simulink model "Battery_Model"  (R2019b)
settings: configuration reference "BMS_Sw_CodeGenConfig" (kept outside this file)
undefined symbols (not defined in the file): Battery, TempInit, ts
libraries: fl_lib x2765, nesl_utility x1565, ee_lib x384, simulink x384, BatteryPack_lib x3
(part 1 of 33)
settings Model: DataDictionary=DD_Battery.sldd  EnableAccessToBaseWorkspace=off  Creator=mluethy  LastModifiedBy=ZHOU Jinhan
settings ConfigSetRef: SourceName=BMS_Sw_CodeGenConfig

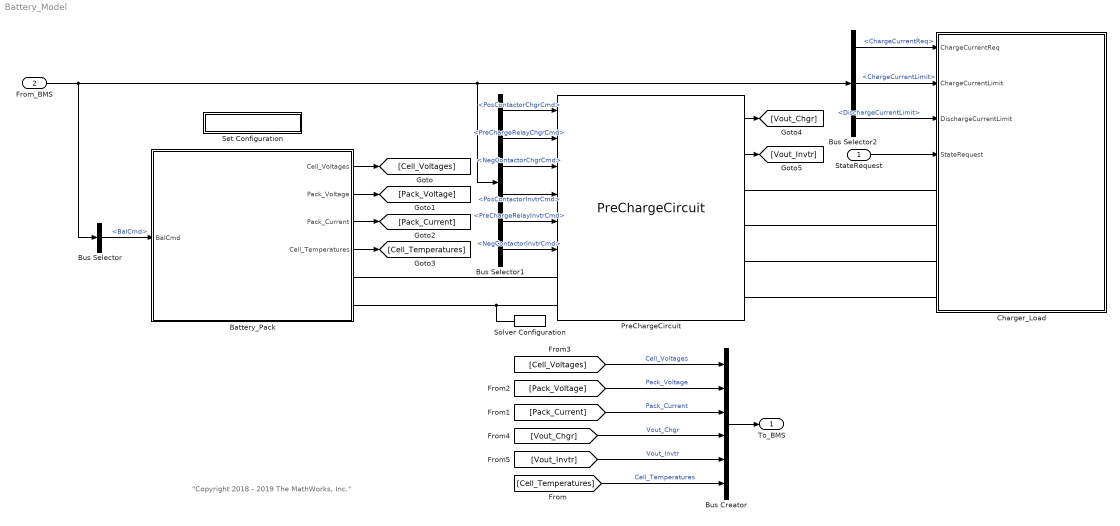
== system Battery_Model ==
  note: "Copyright 2018 - 2019 The MathWorks, Inc."
  StateRequest : Inport  OutDataTypeStr=Enum: SRE  SampleTime=[ts,0]  Interpolate=off
  From_BMS : Inport  Port=2  OutDataTypeStr=Bus: BMS_Output
  Battery_Pack : Subsystem  Variant=on  VariantControl=Variant1
      mask Display: image('Plant_Battery.jpg',[40,65,120,70])
  Bus Selector : BusSelector  OutputSignals=BalCmd
  Bus Selector1 : BusSelector  OutputSignals=PosContactorChgrCmd,PreChargeRelayChgrCmd,NegContactorChgrCmd,PosContactorInvtrCmd,PreChargeRelayInvtrCmd,NegContactorInvtrCmd
  Bus Selector2 : BusSelector  OutputSignals=ChargeCurrentReq,ChargeCurrentLimit,DischargeCurrentLimit
  Bus Creator : BusCreator  Inputs=6  OutDataTypeStr=Bus: BMS_Input  NonVirtualBus=on
  Charger_Load : Subsystem
      mask Display: image('Charger_Load3.jpg',[40,5,150,200])
  PreChargeCircuit : BatteryPack_lib/PreChargeCircuit  SystemSampleTime=-1  Latency=0  AutoFrameSizeCalculation=off
      mask Display: image('PowerElectronics.jpg',[110,60,100,100])
  Set Configuration : Subsystem
      mask Display: disp('Set Plant Configuration');
  Solver Configuration : nesl_utility/Solver Configuration  PhysicalDomain=network_engine_domain  SubClassName=solver  LeftPortType=input  RightPortType=generic  Tones=[]  Harmonics=[]  SimulateNoise=off  Profile=off  UseLocalSampling=off  EnableSwitchedLinearOptims=on  FrequencyDomain=off  UseCCode=off  RelTol=0.001  AbsTol=1e-06  MinStep=1e-09  ToWorkspace=off  RevertToSquareIcSolve=off  NumHomotopyIterations=100  PhasorMode=off  PhasorModeNumHarmonics=1  DoDC=off  ResidualTolerance=1e-09  UseLocalSolver=on  LocalSolverChoice=NE_BACKWARD_EULER_ADVANCER  LocalSolverSampleTime=ts  DoFixedCost=on  MaxNonlinIter=3  MaxModeIter=2  LinearAlgebra=auto  EquationFormulation=NE_TIME_EF  DelaysMemoryBudget=1024  AutomaticFiltering=on  FilteringTimeConstant=0.001  PartitionStorageMethod=AS_NEEDED  PartitionMemoryBudget=1024  PartitionMethod=FAST
  To_BMS : Outport  OutDataTypeStr=Bus: BMS_Input  VectorParamsAs1DForOutWhenUnconnected=off
  wires:
  Bus Selector1/3 -> PreChargeCircuit/3  "<NegContactorChgrCmd>"
  Battery_Pack/2(Pack_Voltage) -> [Pack_Voltage]
  Bus Selector1/6 -> PreChargeCircuit/6  "<NegContactorInvtrCmd>"
  Bus Selector2/3 -> Charger_Load/3(DischargeCurrentLimit)  "<DischargeCurrentLimit>"
  Bus Selector2/1 -> Charger_Load/1(ChargeCurrentReq)  "<ChargeCurrentReq>"
  Battery_Pack/4(Cell_Temperatures) -> [Cell_Temperatures]
  Bus Selector1/1 -> PreChargeCircuit/1  "<PosContactorChgrCmd>"
  [Cell_Temperatures] -> Bus Creator/6  "Cell_Temperatures"
  Bus Selector/1 -> Battery_Pack/1(BalCmd)  "<BalCmd>"
  StateRequest/1 -> Charger_Load/4(StateRequest)
  Battery_Pack/1(Cell_Voltages) -> [Cell_Voltages]
  Bus Selector1/5 -> PreChargeCircuit/5  "<PreChargeRelayInvtrCmd>"
  [Vout_Chgr] -> Bus Creator/4  "Vout_Chgr"
  [Pack_Voltage] -> Bus Creator/2  "Pack_Voltage"
  Bus Selector2/2 -> Charger_Load/2(ChargeCurrentLimit)  "<ChargeCurrentLimit>"
  PreChargeCircuit/2 -> [Vout_Invtr]
  Bus Creator/1 -> To_BMS/1
  [Vout_Invtr] -> Bus Creator/5  "Vout_Invtr"
  Battery_Pack/3(Pack_Current) -> [Pack_Current]
  [Cell_Voltages] -> Bus Creator/1  "Cell_Voltages"
  From_BMS/1 -> Bus Selector1/1, Bus Selector2/1, Bus Selector/1
  PreChargeCircuit/1 -> [Vout_Chgr]
  Bus Selector1/2 -> PreChargeCircuit/2  "<PreChargeRelayChgrCmd>"
  Bus Selector1/4 -> PreChargeCircuit/4  "<PosContactorInvtrCmd>"
  [Pack_Current] -> Bus Creator/3  "Pack_Current"
  connections:
  Battery_Pack/RConn2 -- Solver Configuration/RConn1 -- PreChargeCircuit/LConn2
  Charger_Load/LConn4 -- PreChargeCircuit/RConn4
  PreChargeCircuit/RConn2 -- Charger_Load/LConn2
  Charger_Load/LConn3 -- PreChargeCircuit/RConn3
  PreChargeCircuit/RConn1 -- Charger_Load/LConn1
  Battery_Pack/RConn1 -- PreChargeCircuit/LConn1

== system Battery_Model/Battery_Pack ==
  BalCmd : Inport
  Battery_Pack_1Module : Subsystem  VariantControl=NumModules == 1
  Battery_Pack_7Modules : Subsystem  VariantControl=Choice
  +Batt : PMIOPort  Side=Right
  -Batt : PMIOPort  Port=2  Side=Right
  Cell_Voltages : Outport  VectorParamsAs1DForOutWhenUnconnected=off
  Pack_Voltage : Outport  Port=2  VectorParamsAs1DForOutWhenUnconnected=off
  Pack_Current : Outport  Port=3  VectorParamsAs1DForOutWhenUnconnected=off
  Cell_Temperatures : Outport  Port=4  VectorParamsAs1DForOutWhenUnconnected=off

== system Battery_Model/Charger_Load ==
  ChargeCurrentReq : Inport
  ChargeCurrentLimit : Inport  Port=2
  DischargeCurrentLimit : Inport  Port=3
  StateRequest : Inport  Port=4
  Charger : BatteryPack_lib/Charger  SystemSampleTime=-1  Latency=0  AutoFrameSizeCalculation=off
      mask Display: image('Charger.jpg',[60,35,90,90])
  Data Type Conversion : DataTypeConversion  OutDataTypeStr=int8
  DriveLoad : BatteryPack_lib/DriveLoad  SystemSampleTime=-1  Latency=0  AutoFrameSizeCalculation=off
      mask Display: image('Load.jpg',[60,35,90,90])
  +Chgr : PMIOPort  Side=Left
  -Chgr : PMIOPort  Port=2  Side=Left
  +Invtr : PMIOPort  Port=3  Side=Left
  -Invtr : PMIOPort  Port=4  Side=Left
  wires:
  ChargeCurrentReq/1 -> Charger/1
  Data Type Conversion/1 -> DriveLoad/3, Charger/2
  StateRequest/1 -> Data Type Conversion/1
  DischargeCurrentLimit/1 -> DriveLoad/2
  ChargeCurrentLimit/1 -> DriveLoad/1
  connections:
  DriveLoad/LConn1 -- +Invtr/RConn1
  +Chgr/RConn1 -- Charger/LConn1
  DriveLoad/LConn2 -- -Invtr/RConn1
  -Chgr/RConn1 -- Charger/LConn2

== system Battery_Model/Set Configuration ==
  Battery 1 pack 1RC : Subsystem
      settings: OpenFcn=|
      | SharedDictionaryObj = Simulink.data.dictionary.open('Shared_DD.sldd');
      | try removeDataSource(SharedDictionaryObj,'Battery_1Pack_1RC.sldd')
      | end
      | try removeDataSource(SharedDictionaryObj,'Battery_16Packs_1RC.sldd')
      | end
      | addDataSource(SharedDictionaryObj,'Battery_1Pack_1RC.sldd')
  Battery 7 packs 1RC : Subsystem
      settings: OpenFcn=|
      | SharedDictionaryObj = Simulink.data.dictionary.open('Shared_DD.sldd');
      | try removeDataSource(SharedDictionaryObj,'Battery_1Pack_1RC.sldd')
      | end
      | try removeDataSource(SharedDictionaryObj,'Battery_16Packs_1RC.sldd')
      | end
      | addDataSource(SharedDictionaryObj,'Battery_16Packs_1RC.sldd')

== system Battery_Model/Battery_Pack/Battery_Pack_1Module ==
  BalCmd : Inport
  Cell_3p : Subsystem
  Current Sensor : fl_lib/Electrical/Electrical Sensors/Current Sensor
  Data Type Conversion : DataTypeConversion  OutDataTypeStr=single
  Data Type Conversion1 : DataTypeConversion  OutDataTypeStr=single
  Electrical Reference : fl_lib/Electrical/Electrical Elements/Electrical Reference
  PS-Simulink Converter3 : nesl_utility/PS-Simulink Converter  PhysicalDomain=network_engine_domain  SubClassName=ps_output  LeftPortType=input  RightPortType=output  PseudoPeriodic=off  Frequencies=[]  Unit=V  AffineConversion=off
  PS-Simulink Converter5 : nesl_utility/PS-Simulink Converter  PhysicalDomain=network_engine_domain  SubClassName=ps_output  LeftPortType=input  RightPortType=output  PseudoPeriodic=off  Frequencies=[]  Unit=A  AffineConversion=off
  Voltage Sensor4 : fl_lib/Electrical/Electrical Sensors/Voltage Sensor
  +Batt : PMIOPort  Side=Right
  -Batt : PMIOPort  Port=2  Side=Right
  Pack_Voltage : Outport  VectorParamsAs1DForOutWhenUnconnected=off
  Pack_Current : Outport  Port=2  VectorParamsAs1DForOutWhenUnconnected=off
  Cell_Voltages : Outport  Port=3  VectorParamsAs1DForOutWhenUnconnected=off
  Cell_Temperatures : Outport  Port=4  VectorParamsAs1DForOutWhenUnconnected=off
  wires:
  Data Type Conversion/1 -> Pack_Voltage/1
  Data Type Conversion1/1 -> Pack_Current/1
  PS-Simulink Converter5/1 -> Data Type Conversion1/1
  PS-Simulink Converter3/1 -> Data Type Conversion/1
  BalCmd/1 -> Cell_3p/1(BalCmd)
  Cell_3p/1(Cell_Voltages) -> Cell_Voltages/1
  Cell_3p/2(Cell_Temperatures) -> Cell_Temperatures/1
  connections:
  Electrical Reference/LConn1 -- Voltage Sensor4/RConn2 -- Current Sensor/RConn2 -- -Batt/RConn1
  Voltage Sensor4/RConn1 -- PS-Simulink Converter3/LConn1
  Current Sensor/RConn1 -- PS-Simulink Converter5/LConn1
  Voltage Sensor4/LConn1 -- +Batt/RConn1 -- Cell_3p/RConn1
  Current Sensor/LConn1 -- Cell_3p/RConn2

== system Battery_Model/Battery_Pack/Battery_Pack_7Modules ==
  BalCmd : Inport
  Cell_3p01 : Subsystem
  Cell_3p02 : Subsystem
  Cell_3p03 : Subsystem
  Cell_3p04 : Subsystem
  Cell_3p05 : Subsystem
  Cell_3p06 : Subsystem
  Cell_3p1 : Subsystem
  Constant : Constant  Value=Battery.TempInit  SampleTime=ts
  Current Sensor1 : fl_lib/Electrical/Electrical Sensors/Current Sensor
  Data Type Conversion2 : DataTypeConversion  OutDataTypeStr=double
  Data Type Conversion3 : DataTypeConversion  OutDataTypeStr=single
  Data Type Conversion4 : DataTypeConversion  OutDataTypeStr=single
  PS-Simulink Converter1 : nesl_utility/PS-Simulink Converter  PhysicalDomain=network_engine_domain  SubClassName=ps_output  LeftPortType=input  RightPortType=output  PseudoPeriodic=off  Frequencies=[]  Unit=V  AffineConversion=off
  PS-Simulink Converter2 : nesl_utility/PS-Simulink Converter  PhysicalDomain=network_engine_domain  SubClassName=ps_output  LeftPortType=input  RightPortType=output  PseudoPeriodic=off  Frequencies=[]  Unit=A  AffineConversion=off
  Selector : Selector  InputPortWidth=96  IndexOptions=Starting index (dialog)  Indices=[1]  OutputSizes=6
  Vector Concatenate : Concatenate  NumInputs=7
  Vector Concatenate1 : Concatenate  NumInputs=7
  Voltage Sensor1 : fl_lib/Electrical/Electrical Sensors/Voltage Sensor
  +Batt : PMIOPort  Side=Right
  -Batt : PMIOPort  Port=2  Side=Right
  Cell_Voltages : Outport  VectorParamsAs1DForOutWhenUnconnected=off
  Cell_Temperatures : Outport  Port=2  VectorParamsAs1DForOutWhenUnconnected=off
  Pack_Voltage : Outport  Port=3  VectorParamsAs1DForOutWhenUnconnected=off
  Pack_Current : Outport  Port=4  VectorParamsAs1DForOutWhenUnconnected=off
  wires:
  BalCmd/1 -> Data Type Conversion2/1
  [Module06_Volts] -> Vector Concatenate/6  "Module06_Volts"
  [Module07_Temps] -> Vector Concatenate1/7
  Cell_3p01/2(Cell_Temperatures) -> [Module01_Temps]
  [Module07_Volts] -> Vector Concatenate/7  "Module07_Volts"
  Cell_3p01/1(Cell_Voltages) -> [Module01_Volts]
  [Module01_Temps] -> Vector Concatenate1/1
  [Module02_Volts] -> Vector Concatenate/2  "Module02_Volts"
  [Module02_Temps] -> Vector Concatenate1/2
  [Module06_Temps] -> Vector Concatenate1/6
  Vector Concatenate/1 -> Cell_Voltages/1
  [Module03_Volts] -> Vector Concatenate/3  "Module03_Volts"
  [Module01_Volts] -> Vector Concatenate/1  "Module01_Volts"
  [Module05_Temps] -> Vector Concatenate1/5
  [Module04_Temps] -> Vector Concatenate1/4
  Vector Concatenate1/1 -> Cell_Temperatures/1
  [Module03_Temps] -> Vector Concatenate1/3
  [Module05_Volts] -> Vector Concatenate/5  "Module05_Volts"
  [Module04_Volts] -> Vector Concatenate/4  "Module04_Volts"
  Cell_3p02/1(Cell_Voltages) -> [Module02_Volts]
  Cell_3p02/2(Cell_Temperatures) -> [Module02_Temps]
  Cell_3p03/2(Cell_Temperatures) -> [Module03_Temps]
  Cell_3p03/1(Cell_Voltages) -> [Module03_Volts]
  Cell_3p04/2(Cell_Temperatures) -> [Module04_Temps]
  Cell_3p04/1(Cell_Voltages) -> [Module04_Volts]
  Cell_3p06/2(Cell_Temperatures) -> [Module06_Temps]
  Cell_3p06/1(Cell_Voltages) -> [Module06_Volts]
  Cell_3p05/1(Cell_Voltages) -> [Module05_Volts]
  Cell_3p05/2(Cell_Temperatures) -> [Module05_Temps]
  Cell_3p1/1(Cell_Voltages) -> [Module06_Volts]
  Cell_3p1/2(Cell_Temperatures) -> [Module06_Temps]
  Selector/1 -> Cell_3p06/1(BalCmd), Cell_3p1/1(BalCmd), Cell_3p05/1(BalCmd), Cell_3p04/1(BalCmd), Cell_3p03/1(BalCmd), Cell_3p02/1(BalCmd), Cell_3p01/1(BalCmd)
  Constant/1 -> Cell_3p06/2(AmTmp), Cell_3p1/2(AmTmp), Cell_3p05/2(AmTmp), Cell_3p01/2(AmTmp), Cell_3p02/2(AmTmp), Cell_3p03/2(AmTmp), Cell_3p04/2(AmTmp)
  Data Type Conversion4/1 -> Pack_Current/1
  PS-Simulink Converter1/1 -> Data Type Conversion3/1  "Pack_Voltage"
  Data Type Conversion3/1 -> Pack_Voltage/1
  PS-Simulink Converter2/1 -> Data Type Conversion4/1  "Pack_Current"
  Data Type Conversion2/1 -> Selector/1
  connections:
  Voltage Sensor1/LConn1 -- Cell_3p01/RConn1 -- +Batt/RConn1
  Cell_3p02/RConn1 -- Cell_3p01/RConn2
  Cell_3p03/RConn1 -- Cell_3p02/RConn2
  Cell_3p04/RConn1 -- Cell_3p03/RConn2
  Cell_3p06/RConn1 -- Cell_3p05/RConn2
  Voltage Sensor1/RConn2 -- Cell_3p04/RConn2 -- Cell_3p05/RConn1 -- Current Sensor1/LConn1
  Cell_3p06/RConn2 -- Cell_3p1/RConn1
  PS-Simulink Converter2/LConn1 -- Current Sensor1/RConn1
  -Batt/RConn1 -- Current Sensor1/RConn2
  Voltage Sensor1/RConn1 -- PS-Simulink Converter1/LConn1

== system Battery_Model/Set Configuration/Battery 1 pack 1RC ==

== system Battery_Model/Set Configuration/Battery 7 packs 1RC ==

== system Battery_Model/Battery_Pack/Battery_Pack_1Module/Cell_3p ==
  BalCmd : Inport
  CellMonitoringUnit_1 : Subsystem
  CellMonitoringUnit_2 : Subsystem
  CellMonitoringUnit_3 : Subsystem
  Cell_Module_1 : Subsystem
  Cell_Module_2 : Subsystem
  Cell_Module_3 : Subsystem
  Constant : Constant  Value=TempInit  SampleTime=ts
  Data Type Conversion2 : DataTypeConversion  OutDataTypeStr=double
  Data Type Conversion3 : DataTypeConversion  OutDataTypeStr=single
  Data Type Conversion4 : DataTypeConversion  OutDataTypeStr=single
  Data Type Conversion5 : DataTypeConversion  OutDataTypeStr=single
  Vector Concatenate : Concatenate  NumInputs=3
  Vector Concatenate1 : Concatenate  NumInputs=3
  Cell+ : PMIOPort  Side=Right
  Cell- : PMIOPort  Port=2  Side=Right
  Cell_Voltages : Outport  VectorParamsAs1DForOutWhenUnconnected=off
  Cell_Temperatures : Outport  Port=2  VectorParamsAs1DForOutWhenUnconnected=off
  wires:
  Data Type Conversion4/1 -> [Module01_Volts]
  CellMonitoringUnit_1/1(CellVoltages) -> Data Type Conversion4/1
  Data Type Conversion2/1 -> CellMonitoringUnit_3/1(BalCmd), CellMonitoringUnit_2/1(BalCmd), CellMonitoringUnit_1/1(BalCmd)
  [Module01_Volts] -> Vector Concatenate/1  "Module01_Volts"
  Data Type Conversion5/1 -> [Module03_Volts]
  Constant/1 -> Cell_Module_3/1(AmbientTemp), Cell_Module_2/1(AmbientTemp), Cell_Module_1/1(AmbientTemp)
  CellMonitoringUnit_2/1(CellVoltages) -> Data Type Conversion3/1
  Data Type Conversion3/1 -> [Module02_Volts]
  Cell_Module_1/1(CellTemp) -> [Module01_Temps]
  Cell_Module_2/1(CellTemp) -> [Module02_Temps]
  BalCmd/1 -> Data Type Conversion2/1
  CellMonitoringUnit_3/1(CellVoltages) -> Data Type Conversion5/1
  [Module03_Volts] -> Vector Concatenate/3  "Module03_Volts"
  Vector Concatenate/1 -> Cell_Voltages/1
  [Module02_Volts] -> Vector Concatenate/2  "Module02_Volts"
  Cell_Module_3/1(CellTemp) -> [Module03_Temps]
  [Module03_Temps] -> Vector Concatenate1/3
  [Module01_Temps] -> Vector Concatenate1/1
  [Module02_Temps] -> Vector Concatenate1/2
  Vector Concatenate1/1 -> Cell_Temperatures/1
  connections:
  CellMonitoringUnit_1/LConn9 -- Cell_Module_1/RConn9
  Cell_Module_3/RConn6 -- CellMonitoringUnit_3/LConn6
  Cell_Module_2/RConn11 -- CellMonitoringUnit_2/LConn11
  Cell_Module_3/RConn9 -- CellMonitoringUnit_3/LConn9
  Cell_Module_2/RConn5 -- CellMonitoringUnit_2/LConn5
  CellMonitoringUnit_1/LConn13 -- Cell_Module_1/RConn13
  Cell_Module_2/RConn6 -- CellMonitoringUnit_2/LConn6
  Cell_Module_3/RConn17 -- CellMonitoringUnit_3/LConn17 -- CellMonitoringUnit_2/LConn17 -- Cell-/RConn1 -- CellMonitoringUnit_1/LConn17 -- Cell_Module_1/RConn17 -- Cell_Module_2/RConn17
  CellMonitoringUnit_1/LConn8 -- Cell_Module_1/RConn8
  Cell_Module_2/RConn13 -- CellMonitoringUnit_2/LConn13
  Cell_Module_2/RConn8 -- CellMonitoringUnit_2/LConn8
  CellMonitoringUnit_3/LConn1 -- Cell_Module_3/RConn1 -- Cell_Module_2/RConn1 -- CellMonitoringUnit_2/LConn1 -- CellMonitoringUnit_1/LConn1 -- Cell+/RConn1 -- Cell_Module_1/RConn1
  CellMonitoringUnit_1/LConn7 -- Cell_Module_1/RConn7
  Cell_Module_2/RConn10 -- CellMonitoringUnit_2/LConn10
  Cell_Module_3/RConn3 -- CellMonitoringUnit_3/LConn3
  Cell_Module_2/RConn14 -- CellMonitoringUnit_2/LConn14
  Cell_Module_2/RConn16 -- CellMonitoringUnit_2/LConn16
  Cell_Module_2/RConn12 -- CellMonitoringUnit_2/LConn12
  Cell_Module_2/RConn2 -- CellMonitoringUnit_2/LConn2
  Cell_Module_3/RConn4 -- CellMonitoringUnit_3/LConn4
  Cell_Module_3/RConn2 -- CellMonitoringUnit_3/LConn2
  Cell_Module_3/RConn8 -- CellMonitoringUnit_3/LConn8
  CellMonitoringUnit_1/LConn11 -- Cell_Module_1/RConn11
  Cell_Module_2/RConn9 -- CellMonitoringUnit_2/LConn9
  Cell_Module_3/RConn12 -- CellMonitoringUnit_3/LConn12
  CellMonitoringUnit_1/LConn3 -- Cell_Module_1/RConn3
  CellMonitoringUnit_1/LConn15 -- Cell_Module_1/RConn15
  Cell_Module_3/RConn7 -- CellMonitoringUnit_3/LConn7
  CellMonitoringUnit_1/LConn5 -- Cell_Module_1/RConn5
  Cell_Module_3/RConn15 -- CellMonitoringUnit_3/LConn15
  CellMonitoringUnit_1/LConn12 -- Cell_Module_1/RConn12
  CellMonitoringUnit_1/LConn10 -- Cell_Module_1/RConn10
  Cell_Module_2/RConn3 -- CellMonitoringUnit_2/LConn3
  CellMonitoringUnit_1/LConn6 -- Cell_Module_1/RConn6
  Cell_Module_2/RConn4 -- CellMonitoringUnit_2/LConn4
  Cell_Module_3/RConn10 -- CellMonitoringUnit_3/LConn10
  CellMonitoringUnit_1/LConn14 -- Cell_Module_1/RConn14
  CellMonitoringUnit_1/LConn4 -- Cell_Module_1/RConn4
  Cell_Module_3/RConn16 -- CellMonitoringUnit_3/LConn16
  Cell_Module_3/RConn11 -- CellMonitoringUnit_3/LConn11
  Cell_Module_3/RConn13 -- CellMonitoringUnit_3/LConn13
  Cell_Module_3/RConn14 -- CellMonitoringUnit_3/LConn14
  Cell_Module_3/RConn5 -- CellMonitoringUnit_3/LConn5
  Cell_Module_2/RConn15 -- CellMonitoringUnit_2/LConn15
  Cell_Module_2/RConn7 -- CellMonitoringUnit_2/LConn7
  CellMonitoringUnit_1/LConn2 -- Cell_Module_1/RConn2
  CellMonitoringUnit_1/LConn16 -- Cell_Module_1/RConn16

== system Battery_Model/Battery_Pack/Battery_Pack_7Modules/Cell_3p01 ==
  BalCmd : Inport
  AmTmp : Inport  Port=2
  CellMonitoringUnit_1 : Subsystem
  CellMonitoringUnit_2 : Subsystem
  CellMonitoringUnit_3 : Subsystem
  Cell_Module_1 : Subsystem
  Cell_Module_2 : Subsystem
  Cell_Module_3 : Subsystem
  Data Type Conversion2 : DataTypeConversion  OutDataTypeStr=double
  Data Type Conversion3 : DataTypeConversion  OutDataTypeStr=single
  Data Type Conversion4 : DataTypeConversion  OutDataTypeStr=single
  Data Type Conversion5 : DataTypeConversion  OutDataTypeStr=single
  Vector Concatenate : Concatenate  NumInputs=3
  Vector Concatenate1 : Concatenate  NumInputs=3
  Cell+ : PMIOPort  Side=Right
  Cell- : PMIOPort  Port=2  Side=Right
  Cell_Voltages : Outport  VectorParamsAs1DForOutWhenUnconnected=off
  Cell_Temperatures : Outport  Port=2  VectorParamsAs1DForOutWhenUnconnected=off
  wires:
  Data Type Conversion4/1 -> [Module01_Volts]
  CellMonitoringUnit_1/1(CellVoltages) -> Data Type Conversion4/1
  Data Type Conversion2/1 -> CellMonitoringUnit_3/1(BalCmd), CellMonitoringUnit_2/1(BalCmd), CellMonitoringUnit_1/1(BalCmd)
  [Module01_Volts] -> Vector Concatenate/1  "Module01_Volts"
  Data Type Conversion5/1 -> [Module03_Volts]
  AmTmp/1 -> Cell_Module_3/1(AmbientTemp), Cell_Module_2/1(AmbientTemp), Cell_Module_1/1(AmbientTemp)
  CellMonitoringUnit_2/1(CellVoltages) -> Data Type Conversion3/1
  Data Type Conversion3/1 -> [Module02_Volts]
  Cell_Module_1/1(CellTemp) -> [Module01_Temps]
  Cell_Module_2/1(CellTemp) -> [Module02_Temps]
  BalCmd/1 -> Data Type Conversion2/1
  CellMonitoringUnit_3/1(CellVoltages) -> Data Type Conversion5/1
  [Module03_Volts] -> Vector Concatenate/3  "Module03_Volts"
  Vector Concatenate/1 -> Cell_Voltages/1
  [Module02_Volts] -> Vector Concatenate/2  "Module02_Volts"
  Cell_Module_3/1(CellTemp) -> [Module03_Temps]
  [Module03_Temps] -> Vector Concatenate1/3
  [Module01_Temps] -> Vector Concatenate1/1
  [Module02_Temps] -> Vector Concatenate1/2
  Vector Concatenate1/1 -> Cell_Temperatures/1
  connections:
  CellMonitoringUnit_1/LConn9 -- Cell_Module_1/RConn9
  Cell_Module_3/RConn6 -- CellMonitoringUnit_3/LConn6
  Cell_Module_2/RConn11 -- CellMonitoringUnit_2/LConn11
  Cell_Module_3/RConn9 -- CellMonitoringUnit_3/LConn9
  Cell_Module_2/RConn5 -- CellMonitoringUnit_2/LConn5
  CellMonitoringUnit_1/LConn13 -- Cell_Module_1/RConn13
  Cell_Module_2/RConn6 -- CellMonitoringUnit_2/LConn6
  Cell_Module_1/RConn17 -- Cell-/RConn1 -- CellMonitoringUnit_2/LConn17 -- CellMonitoringUnit_3/LConn17 -- Cell_Module_3/RConn17 -- Cell_Module_2/RConn17 -- CellMonitoringUnit_1/LConn17
  CellMonitoringUnit_1/LConn8 -- Cell_Module_1/RConn8
  Cell_Module_2/RConn13 -- CellMonitoringUnit_2/LConn13
  Cell_Module_2/RConn8 -- CellMonitoringUnit_2/LConn8
  CellMonitoringUnit_1/LConn1 -- Cell_Module_3/RConn1 -- CellMonitoringUnit_3/LConn1 -- Cell_Module_2/RConn1 -- CellMonitoringUnit_2/LConn1 -- Cell_Module_1/RConn1 -- Cell+/RConn1
  CellMonitoringUnit_1/LConn7 -- Cell_Module_1/RConn7
  Cell_Module_2/RConn10 -- CellMonitoringUnit_2/LConn10
  Cell_Module_3/RConn3 -- CellMonitoringUnit_3/LConn3
  Cell_Module_2/RConn14 -- CellMonitoringUnit_2/LConn14
  Cell_Module_2/RConn16 -- CellMonitoringUnit_2/LConn16
  Cell_Module_2/RConn12 -- CellMonitoringUnit_2/LConn12
  Cell_Module_2/RConn2 -- CellMonitoringUnit_2/LConn2
  Cell_Module_3/RConn4 -- CellMonitoringUnit_3/LConn4
  Cell_Module_3/RConn2 -- CellMonitoringUnit_3/LConn2
  Cell_Module_3/RConn8 -- CellMonitoringUnit_3/LConn8
  CellMonitoringUnit_1/LConn11 -- Cell_Module_1/RConn11
  Cell_Module_2/RConn9 -- CellMonitoringUnit_2/LConn9
  Cell_Module_3/RConn12 -- CellMonitoringUnit_3/LConn12
  CellMonitoringUnit_1/LConn3 -- Cell_Module_1/RConn3
  CellMonitoringUnit_1/LConn15 -- Cell_Module_1/RConn15
  Cell_Module_3/RConn7 -- CellMonitoringUnit_3/LConn7
  CellMonitoringUnit_1/LConn5 -- Cell_Module_1/RConn5
  Cell_Module_3/RConn15 -- CellMonitoringUnit_3/LConn15
  CellMonitoringUnit_1/LConn12 -- Cell_Module_1/RConn12
  CellMonitoringUnit_1/LConn10 -- Cell_Module_1/RConn10
  Cell_Module_2/RConn3 -- CellMonitoringUnit_2/LConn3
  CellMonitoringUnit_1/LConn6 -- Cell_Module_1/RConn6
  Cell_Module_2/RConn4 -- CellMonitoringUnit_2/LConn4
  Cell_Module_3/RConn10 -- CellMonitoringUnit_3/LConn10
  CellMonitoringUnit_1/LConn14 -- Cell_Module_1/RConn14
  CellMonitoringUnit_1/LConn4 -- Cell_Module_1/RConn4
  Cell_Module_3/RConn16 -- CellMonitoringUnit_3/LConn16
  Cell_Module_3/RConn11 -- CellMonitoringUnit_3/LConn11
  Cell_Module_3/RConn13 -- CellMonitoringUnit_3/LConn13
  Cell_Module_3/RConn14 -- CellMonitoringUnit_3/LConn14
  Cell_Module_3/RConn5 -- CellMonitoringUnit_3/LConn5
  Cell_Module_2/RConn15 -- CellMonitoringUnit_2/LConn15
  Cell_Module_2/RConn7 -- CellMonitoringUnit_2/LConn7
  CellMonitoringUnit_1/LConn2 -- Cell_Module_1/RConn2
  CellMonitoringUnit_1/LConn16 -- Cell_Module_1/RConn16

== system Battery_Model/Battery_Pack/Battery_Pack_7Modules/Cell_3p02 ==
  BalCmd : Inport
  AmTmp : Inport  Port=2
  CellMonitoringUnit_1 : Subsystem
  CellMonitoringUnit_2 : Subsystem
  CellMonitoringUnit_3 : Subsystem
  Cell_Module_1 : Subsystem
  Cell_Module_2 : Subsystem
  Cell_Module_3 : Subsystem
  Data Type Conversion2 : DataTypeConversion  OutDataTypeStr=double
  Data Type Conversion3 : DataTypeConversion  OutDataTypeStr=single
  Data Type Conversion4 : DataTypeConversion  OutDataTypeStr=single
  Data Type Conversion5 : DataTypeConversion  OutDataTypeStr=single
  Vector Concatenate : Concatenate  NumInputs=3
  Vector Concatenate1 : Concatenate  NumInputs=3
  Cell+ : PMIOPort  Side=Right
  Cell- : PMIOPort  Port=2  Side=Right
  Cell_Voltages : Outport  VectorParamsAs1DForOutWhenUnconnected=off
  Cell_Temperatures : Outport  Port=2  VectorParamsAs1DForOutWhenUnconnected=off
  wires:
  Data Type Conversion4/1 -> [Module01_Volts]
  CellMonitoringUnit_1/1(CellVoltages) -> Data Type Conversion4/1
  Data Type Conversion2/1 -> CellMonitoringUnit_3/1(BalCmd), CellMonitoringUnit_2/1(BalCmd), CellMonitoringUnit_1/1(BalCmd)
  [Module01_Volts] -> Vector Concatenate/1  "Module01_Volts"
  Data Type Conversion5/1 -> [Module03_Volts]
  AmTmp/1 -> Cell_Module_3/1(AmbientTemp), Cell_Module_2/1(AmbientTemp), Cell_Module_1/1(AmbientTemp)
  CellMonitoringUnit_2/1(CellVoltages) -> Data Type Conversion3/1
  Data Type Conversion3/1 -> [Module02_Volts]
  Cell_Module_1/1(CellTemp) -> [Module01_Temps]
  Cell_Module_2/1(CellTemp) -> [Module02_Temps]
  BalCmd/1 -> Data Type Conversion2/1
  CellMonitoringUnit_3/1(CellVoltages) -> Data Type Conversion5/1
  [Module03_Volts] -> Vector Concatenate/3  "Module03_Volts"
  Vector Concatenate/1 -> Cell_Voltages/1
  [Module02_Volts] -> Vector Concatenate/2  "Module02_Volts"
  Cell_Module_3/1(CellTemp) -> [Module03_Temps]
  [Module03_Temps] -> Vector Concatenate1/3
  [Module01_Temps] -> Vector Concatenate1/1
  [Module02_Temps] -> Vector Concatenate1/2
  Vector Concatenate1/1 -> Cell_Temperatures/1
  connections:
  CellMonitoringUnit_1/LConn9 -- Cell_Module_1/RConn9
  Cell_Module_3/RConn6 -- CellMonitoringUnit_3/LConn6
  Cell_Module_2/RConn11 -- CellMonitoringUnit_2/LConn11
  Cell_Module_3/RConn9 -- CellMonitoringUnit_3/LConn9
  Cell_Module_2/RConn5 -- CellMonitoringUnit_2/LConn5
  CellMonitoringUnit_1/LConn13 -- Cell_Module_1/RConn13
  Cell_Module_2/RConn6 -- CellMonitoringUnit_2/LConn6
  Cell_Module_1/RConn17 -- Cell-/RConn1 -- CellMonitoringUnit_2/LConn17 -- CellMonitoringUnit_3/LConn17 -- Cell_Module_3/RConn17 -- Cell_Module_2/RConn17 -- CellMonitoringUnit_1/LConn17
  CellMonitoringUnit_1/LConn8 -- Cell_Module_1/RConn8
  Cell_Module_2/RConn13 -- CellMonitoringUnit_2/LConn13
  Cell_Module_2/RConn8 -- CellMonitoringUnit_2/LConn8
  CellMonitoringUnit_1/LConn1 -- Cell_Module_3/RConn1 -- CellMonitoringUnit_3/LConn1 -- Cell_Module_2/RConn1 -- CellMonitoringUnit_2/LConn1 -- Cell_Module_1/RConn1 -- Cell+/RConn1
  CellMonitoringUnit_1/LConn7 -- Cell_Module_1/RConn7
  Cell_Module_2/RConn10 -- CellMonitoringUnit_2/LConn10
  Cell_Module_3/RConn3 -- CellMonitoringUnit_3/LConn3
  Cell_Module_2/RConn14 -- CellMonitoringUnit_2/LConn14
  Cell_Module_2/RConn16 -- CellMonitoringUnit_2/LConn16
  Cell_Module_2/RConn12 -- CellMonitoringUnit_2/LConn12
  Cell_Module_2/RConn2 -- CellMonitoringUnit_2/LConn2
  Cell_Module_3/RConn4 -- CellMonitoringUnit_3/LConn4
  Cell_Module_3/RConn2 -- CellMonitoringUnit_3/LConn2
  Cell_Module_3/RConn8 -- CellMonitoringUnit_3/LConn8
  CellMonitoringUnit_1/LConn11 -- Cell_Module_1/RConn11
  Cell_Module_2/RConn9 -- CellMonitoringUnit_2/LConn9
  Cell_Module_3/RConn12 -- CellMonitoringUnit_3/LConn12
  CellMonitoringUnit_1/LConn3 -- Cell_Module_1/RConn3
  CellMonitoringUnit_1/LConn15 -- Cell_Module_1/RConn15
  Cell_Module_3/RConn7 -- CellMonitoringUnit_3/LConn7
  CellMonitoringUnit_1/LConn5 -- Cell_Module_1/RConn5
  Cell_Module_3/RConn15 -- CellMonitoringUnit_3/LConn15
  CellMonitoringUnit_1/LConn12 -- Cell_Module_1/RConn12
  CellMonitoringUnit_1/LConn10 -- Cell_Module_1/RConn10
  Cell_Module_2/RConn3 -- CellMonitoringUnit_2/LConn3
  CellMonitoringUnit_1/LConn6 -- Cell_Module_1/RConn6
  Cell_Module_2/RConn4 -- CellMonitoringUnit_2/LConn4
  Cell_Module_3/RConn10 -- CellMonitoringUnit_3/LConn10
  CellMonitoringUnit_1/LConn14 -- Cell_Module_1/RConn14
  CellMonitoringUnit_1/LConn4 -- Cell_Module_1/RConn4
  Cell_Module_3/RConn16 -- CellMonitoringUnit_3/LConn16
  Cell_Module_3/RConn11 -- CellMonitoringUnit_3/LConn11
  Cell_Module_3/RConn13 -- CellMonitoringUnit_3/LConn13
  Cell_Module_3/RConn14 -- CellMonitoringUnit_3/LConn14
  Cell_Module_3/RConn5 -- CellMonitoringUnit_3/LConn5
  Cell_Module_2/RConn15 -- CellMonitoringUnit_2/LConn15
  Cell_Module_2/RConn7 -- CellMonitoringUnit_2/LConn7
  CellMonitoringUnit_1/LConn2 -- Cell_Module_1/RConn2
  CellMonitoringUnit_1/LConn16 -- Cell_Module_1/RConn16

== system Battery_Model/Battery_Pack/Battery_Pack_7Modules/Cell_3p03 ==
  BalCmd : Inport
  AmTmp : Inport  Port=2
  CellMonitoringUnit_1 : Subsystem
  CellMonitoringUnit_2 : Subsystem
  CellMonitoringUnit_3 : Subsystem
  Cell_Module_1 : Subsystem
  Cell_Module_2 : Subsystem
  Cell_Module_3 : Subsystem
  Data Type Conversion2 : DataTypeConversion  OutDataTypeStr=double
  Data Type Conversion3 : DataTypeConversion  OutDataTypeStr=single
  Data Type Conversion4 : DataTypeConversion  OutDataTypeStr=single
  Data Type Conversion5 : DataTypeConversion  OutDataTypeStr=single
  Vector Concatenate : Concatenate  NumInputs=3
  Vector Concatenate1 : Concatenate  NumInputs=3
  Cell+ : PMIOPort  Side=Right
  Cell- : PMIOPort  Port=2  Side=Right
  Cell_Voltages : Outport  VectorParamsAs1DForOutWhenUnconnected=off
  Cell_Temperatures : Outport  Port=2  VectorParamsAs1DForOutWhenUnconnected=off
  wires:
  Data Type Conversion4/1 -> [Module01_Volts]
  CellMonitoringUnit_1/1(CellVoltages) -> Data Type Conversion4/1
  Data Type Conversion2/1 -> CellMonitoringUnit_3/1(BalCmd), CellMonitoringUnit_2/1(BalCmd), CellMonitoringUnit_1/1(BalCmd)
  [Module01_Volts] -> Vector Concatenate/1  "Module01_Volts"
  Data Type Conversion5/1 -> [Module03_Volts]
  AmTmp/1 -> Cell_Module_3/1(AmbientTemp), Cell_Module_2/1(AmbientTemp), Cell_Module_1/1(AmbientTemp)
  CellMonitoringUnit_2/1(CellVoltages) -> Data Type Conversion3/1
  Data Type Conversion3/1 -> [Module02_Volts]
  Cell_Module_1/1(CellTemp) -> [Module01_Temps]
  Cell_Module_2/1(CellTemp) -> [Module02_Temps]
  BalCmd/1 -> Data Type Conversion2/1
  CellMonitoringUnit_3/1(CellVoltages) -> Data Type Conversion5/1
  [Module03_Volts] -> Vector Concatenate/3  "Module03_Volts"
  Vector Concatenate/1 -> Cell_Voltages/1
  [Module02_Volts] -> Vector Concatenate/2  "Module02_Volts"
  Cell_Module_3/1(CellTemp) -> [Module03_Temps]
  [Module03_Temps] -> Vector Concatenate1/3
  [Module01_Temps] -> Vector Concatenate1/1
  [Module02_Temps] -> Vector Concatenate1/2
  Vector Concatenate1/1 -> Cell_Temperatures/1
  connections:
  CellMonitoringUnit_1/LConn9 -- Cell_Module_1/RConn9
  Cell_Module_3/RConn6 -- CellMonitoringUnit_3/LConn6
  Cell_Module_2/RConn11 -- CellMonitoringUnit_2/LConn11
  Cell_Module_3/RConn9 -- CellMonitoringUnit_3/LConn9
  Cell_Module_2/RConn5 -- CellMonitoringUnit_2/LConn5
  CellMonitoringUnit_1/LConn13 -- Cell_Module_1/RConn13
  Cell_Module_2/RConn6 -- CellMonitoringUnit_2/LConn6
  Cell_Module_1/RConn17 -- Cell-/RConn1 -- CellMonitoringUnit_2/LConn17 -- CellMonitoringUnit_3/LConn17 -- Cell_Module_3/RConn17 -- Cell_Module_2/RConn17 -- CellMonitoringUnit_1/LConn17
  CellMonitoringUnit_1/LConn8 -- Cell_Module_1/RConn8
  Cell_Module_2/RConn13 -- CellMonitoringUnit_2/LConn13
  Cell_Module_2/RConn8 -- CellMonitoringUnit_2/LConn8
  CellMonitoringUnit_1/LConn1 -- Cell_Module_3/RConn1 -- CellMonitoringUnit_3/LConn1 -- Cell_Module_2/RConn1 -- CellMonitoringUnit_2/LConn1 -- Cell_Module_1/RConn1 -- Cell+/RConn1
  CellMonitoringUnit_1/LConn7 -- Cell_Module_1/RConn7
  Cell_Module_2/RConn10 -- CellMonitoringUnit_2/LConn10
  Cell_Module_3/RConn3 -- CellMonitoringUnit_3/LConn3
  Cell_Module_2/RConn14 -- CellMonitoringUnit_2/LConn14
  Cell_Module_2/RConn16 -- CellMonitoringUnit_2/LConn16
  Cell_Module_2/RConn12 -- CellMonitoringUnit_2/LConn12
  Cell_Module_2/RConn2 -- CellMonitoringUnit_2/LConn2
  Cell_Module_3/RConn4 -- CellMonitoringUnit_3/LConn4
  Cell_Module_3/RConn2 -- CellMonitoringUnit_3/LConn2
  Cell_Module_3/RConn8 -- CellMonitoringUnit_3/LConn8
  CellMonitoringUnit_1/LConn11 -- Cell_Module_1/RConn11
  Cell_Module_2/RConn9 -- CellMonitoringUnit_2/LConn9
  Cell_Module_3/RConn12 -- CellMonitoringUnit_3/LConn12
  CellMonitoringUnit_1/LConn3 -- Cell_Module_1/RConn3
  CellMonitoringUnit_1/LConn15 -- Cell_Module_1/RConn15
  Cell_Module_3/RConn7 -- CellMonitoringUnit_3/LConn7
  CellMonitoringUnit_1/LConn5 -- Cell_Module_1/RConn5
  Cell_Module_3/RConn15 -- CellMonitoringUnit_3/LConn15
  CellMonitoringUnit_1/LConn12 -- Cell_Module_1/RConn12
  CellMonitoringUnit_1/LConn10 -- Cell_Module_1/RConn10
  Cell_Module_2/RConn3 -- CellMonitoringUnit_2/LConn3
  CellMonitoringUnit_1/LConn6 -- Cell_Module_1/RConn6
  Cell_Module_2/RConn4 -- CellMonitoringUnit_2/LConn4
  Cell_Module_3/RConn10 -- CellMonitoringUnit_3/LConn10
  CellMonitoringUnit_1/LConn14 -- Cell_Module_1/RConn14
  CellMonitoringUnit_1/LConn4 -- Cell_Module_1/RConn4
  Cell_Module_3/RConn16 -- CellMonitoringUnit_3/LConn16
  Cell_Module_3/RConn11 -- CellMonitoringUnit_3/LConn11
  Cell_Module_3/RConn13 -- CellMonitoringUnit_3/LConn13
  Cell_Module_3/RConn14 -- CellMonitoringUnit_3/LConn14
  Cell_Module_3/RConn5 -- CellMonitoringUnit_3/LConn5
  Cell_Module_2/RConn15 -- CellMonitoringUnit_2/LConn15
  Cell_Module_2/RConn7 -- CellMonitoringUnit_2/LConn7
  CellMonitoringUnit_1/LConn2 -- Cell_Module_1/RConn2
  CellMonitoringUnit_1/LConn16 -- Cell_Module_1/RConn16

== system Battery_Model/Battery_Pack/Battery_Pack_7Modules/Cell_3p04 ==
  BalCmd : Inport
  AmTmp : Inport  Port=2
  CellMonitoringUnit_1 : Subsystem
  CellMonitoringUnit_2 : Subsystem
  CellMonitoringUnit_3 : Subsystem
  Cell_Module_1 : Subsystem
  Cell_Module_2 : Subsystem
  Cell_Module_3 : Subsystem
  Data Type Conversion2 : DataTypeConversion  OutDataTypeStr=double
  Data Type Conversion3 : DataTypeConversion  OutDataTypeStr=single
  Data Type Conversion4 : DataTypeConversion  OutDataTypeStr=single
  Data Type Conversion5 : DataTypeConversion  OutDataTypeStr=single
  Vector Concatenate : Concatenate  NumInputs=3
  Vector Concatenate1 : Concatenate  NumInputs=3
  Cell+ : PMIOPort  Side=Right
  Cell- : PMIOPort  Port=2  Side=Right
  Cell_Voltages : Outport  VectorParamsAs1DForOutWhenUnconnected=off
  Cell_Temperatures : Outport  Port=2  VectorParamsAs1DForOutWhenUnconnected=off
  wires:
  Data Type Conversion4/1 -> [Module01_Volts]
  CellMonitoringUnit_1/1(CellVoltages) -> Data Type Conversion4/1
  Data Type Conversion2/1 -> CellMonitoringUnit_3/1(BalCmd), CellMonitoringUnit_2/1(BalCmd), CellMonitoringUnit_1/1(BalCmd)
  [Module01_Volts] -> Vector Concatenate/1  "Module01_Volts"
  Data Type Conversion5/1 -> [Module03_Volts]
  AmTmp/1 -> Cell_Module_3/1(AmbientTemp), Cell_Module_2/1(AmbientTemp), Cell_Module_1/1(AmbientTemp)
  CellMonitoringUnit_2/1(CellVoltages) -> Data Type Conversion3/1
  Data Type Conversion3/1 -> [Module02_Volts]
  Cell_Module_1/1(CellTemp) -> [Module01_Temps]
  Cell_Module_2/1(CellTemp) -> [Module02_Temps]
  BalCmd/1 -> Data Type Conversion2/1
  CellMonitoringUnit_3/1(CellVoltages) -> Data Type Conversion5/1
  [Module03_Volts] -> Vector Concatenate/3  "Module03_Volts"
  Vector Concatenate/1 -> Cell_Voltages/1
  [Module02_Volts] -> Vector Concatenate/2  "Module02_Volts"
  Cell_Module_3/1(CellTemp) -> [Module03_Temps]
  [Module03_Temps] -> Vector Concatenate1/3
  [Module01_Temps] -> Vector Concatenate1/1
  [Module02_Temps] -> Vector Concatenate1/2
  Vector Concatenate1/1 -> Cell_Temperatures/1
  connections:
  CellMonitoringUnit_1/LConn9 -- Cell_Module_1/RConn9
  Cell_Module_3/RConn6 -- CellMonitoringUnit_3/LConn6
  Cell_Module_2/RConn11 -- CellMonitoringUnit_2/LConn11
  Cell_Module_3/RConn9 -- CellMonitoringUnit_3/LConn9
  Cell_Module_2/RConn5 -- CellMonitoringUnit_2/LConn5
  CellMonitoringUnit_1/LConn13 -- Cell_Module_1/RConn13
  Cell_Module_2/RConn6 -- CellMonitoringUnit_2/LConn6
  Cell_Module_1/RConn17 -- Cell-/RConn1 -- CellMonitoringUnit_2/LConn17 -- CellMonitoringUnit_3/LConn17 -- Cell_Module_3/RConn17 -- Cell_Module_2/RConn17 -- CellMonitoringUnit_1/LConn17
  CellMonitoringUnit_1/LConn8 -- Cell_Module_1/RConn8
  Cell_Module_2/RConn13 -- CellMonitoringUnit_2/LConn13
  Cell_Module_2/RConn8 -- CellMonitoringUnit_2/LConn8
  CellMonitoringUnit_1/LConn1 -- Cell_Module_3/RConn1 -- CellMonitoringUnit_3/LConn1 -- Cell_Module_2/RConn1 -- CellMonitoringUnit_2/LConn1 -- Cell_Module_1/RConn1 -- Cell+/RConn1
  CellMonitoringUnit_1/LConn7 -- Cell_Module_1/RConn7
  Cell_Module_2/RConn10 -- CellMonitoringUnit_2/LConn10
  Cell_Module_3/RConn3 -- CellMonitoringUnit_3/LConn3
  Cell_Module_2/RConn14 -- CellMonitoringUnit_2/LConn14
  Cell_Module_2/RConn16 -- CellMonitoringUnit_2/LConn16
  Cell_Module_2/RConn12 -- CellMonitoringUnit_2/LConn12
  Cell_Module_2/RConn2 -- CellMonitoringUnit_2/LConn2
  Cell_Module_3/RConn4 -- CellMonitoringUnit_3/LConn4
  Cell_Module_3/RConn2 -- CellMonitoringUnit_3/LConn2
  Cell_Module_3/RConn8 -- CellMonitoringUnit_3/LConn8
  CellMonitoringUnit_1/LConn11 -- Cell_Module_1/RConn11
  Cell_Module_2/RConn9 -- CellMonitoringUnit_2/LConn9
  Cell_Module_3/RConn12 -- CellMonitoringUnit_3/LConn12
  CellMonitoringUnit_1/LConn3 -- Cell_Module_1/RConn3
  CellMonitoringUnit_1/LConn15 -- Cell_Module_1/RConn15
  Cell_Module_3/RConn7 -- CellMonitoringUnit_3/LConn7
  CellMonitoringUnit_1/LConn5 -- Cell_Module_1/RConn5
  Cell_Module_3/RConn15 -- CellMonitoringUnit_3/LConn15
  CellMonitoringUnit_1/LConn12 -- Cell_Module_1/RConn12
  CellMonitoringUnit_1/LConn10 -- Cell_Module_1/RConn10
  Cell_Module_2/RConn3 -- CellMonitoringUnit_2/LConn3
  CellMonitoringUnit_1/LConn6 -- Cell_Module_1/RConn6
  Cell_Module_2/RConn4 -- CellMonitoringUnit_2/LConn4
  Cell_Module_3/RConn10 -- CellMonitoringUnit_3/LConn10
  CellMonitoringUnit_1/LConn14 -- Cell_Module_1/RConn14
  CellMonitoringUnit_1/LConn4 -- Cell_Module_1/RConn4
  Cell_Module_3/RConn16 -- CellMonitoringUnit_3/LConn16
  Cell_Module_3/RConn11 -- CellMonitoringUnit_3/LConn11
  Cell_Module_3/RConn13 -- CellMonitoringUnit_3/LConn13
  Cell_Module_3/RConn14 -- CellMonitoringUnit_3/LConn14
  Cell_Module_3/RConn5 -- CellMonitoringUnit_3/LConn5
  Cell_Module_2/RConn15 -- CellMonitoringUnit_2/LConn15
  Cell_Module_2/RConn7 -- CellMonitoringUnit_2/LConn7
  CellMonitoringUnit_1/LConn2 -- Cell_Module_1/RConn2
  CellMonitoringUnit_1/LConn16 -- Cell_Module_1/RConn16

== system Battery_Model/Battery_Pack/Battery_Pack_7Modules/Cell_3p05 ==
  BalCmd : Inport
  AmTmp : Inport  Port=2
  CellMonitoringUnit_1 : Subsystem
  CellMonitoringUnit_2 : Subsystem
  CellMonitoringUnit_3 : Subsystem
  Cell_Module_1 : Subsystem
  Cell_Module_2 : Subsystem
  Cell_Module_3 : Subsystem
  Data Type Conversion2 : DataTypeConversion  OutDataTypeStr=double
  Data Type Conversion3 : DataTypeConversion  OutDataTypeStr=single
  Data Type Conversion4 : DataTypeConversion  OutDataTypeStr=single
  Data Type Conversion5 : DataTypeConversion  OutDataTypeStr=single
  Vector Concatenate : Concatenate  NumInputs=3
  Vector Concatenate1 : Concatenate  NumInputs=3
  Cell+ : PMIOPort  Side=Right
  Cell- : PMIOPort  Port=2  Side=Right
  Cell_Voltages : Outport  VectorParamsAs1DForOutWhenUnconnected=off
  Cell_Temperatures : Outport  Port=2  VectorParamsAs1DForOutWhenUnconnected=off
  wires:
  Vector Concatenate1/1 -> Cell_Temperatures/1
  [Module02_Temps] -> Vector Concatenate1/2
  [Module01_Temps] -> Vector Concatenate1/1
  [Module03_Temps] -> Vector Concatenate1/3
  Cell_Module_3/1(CellTemp) -> [Module03_Temps]
  [Module02_Volts] -> Vector Concatenate/2  "Module02_Volts"
  Vector Concatenate/1 -> Cell_Voltages/1
  [Module03_Volts] -> Vector Concatenate/3  "Module03_Volts"
  CellMonitoringUnit_3/1(CellVoltages) -> Data Type Conversion5/1
  BalCmd/1 -> Data Type Conversion2/1
  Cell_Module_2/1(CellTemp) -> [Module02_Temps]
  Cell_Module_1/1(CellTemp) -> [Module01_Temps]
  Data Type Conversion3/1 -> [Module02_Volts]
  CellMonitoringUnit_2/1(CellVoltages) -> Data Type Conversion3/1
  AmTmp/1 -> Cell_Module_1/1(AmbientTemp), Cell_Module_2/1(AmbientTemp), Cell_Module_3/1(AmbientTemp)
  Data Type Conversion5/1 -> [Module03_Volts]
  [Module01_Volts] -> Vector Concatenate/1  "Module01_Volts"
  Data Type Conversion2/1 -> CellMonitoringUnit_1/1(BalCmd), CellMonitoringUnit_2/1(BalCmd), CellMonitoringUnit_3/1(BalCmd)
  CellMonitoringUnit_1/1(CellVoltages) -> Data Type Conversion4/1
  Data Type Conversion4/1 -> [Module01_Volts]
  connections:
  CellMonitoringUnit_1/LConn16 -- Cell_Module_1/RConn16
  CellMonitoringUnit_1/LConn2 -- Cell_Module_1/RConn2
  Cell_Module_2/RConn7 -- CellMonitoringUnit_2/LConn7
  Cell_Module_2/RConn15 -- CellMonitoringUnit_2/LConn15
  Cell_Module_3/RConn5 -- CellMonitoringUnit_3/LConn5
  Cell_Module_3/RConn14 -- CellMonitoringUnit_3/LConn14
  Cell_Module_3/RConn13 -- CellMonitoringUnit_3/LConn13
  Cell_Module_3/RConn11 -- CellMonitoringUnit_3/LConn11
  Cell_Module_3/RConn16 -- CellMonitoringUnit_3/LConn16
  CellMonitoringUnit_1/LConn4 -- Cell_Module_1/RConn4
  CellMonitoringUnit_1/LConn14 -- Cell_Module_1/RConn14
  Cell_Module_3/RConn10 -- CellMonitoringUnit_3/LConn10
  Cell_Module_2/RConn4 -- CellMonitoringUnit_2/LConn4
  CellMonitoringUnit_1/LConn6 -- Cell_Module_1/RConn6
  Cell_Module_2/RConn3 -- CellMonitoringUnit_2/LConn3
  CellMonitoringUnit_1/LConn10 -- Cell_Module_1/RConn10
  CellMonitoringUnit_1/LConn12 -- Cell_Module_1/RConn12
  Cell_Module_3/RConn15 -- CellMonitoringUnit_3/LConn15
  CellMonitoringUnit_1/LConn5 -- Cell_Module_1/RConn5
  Cell_Module_3/RConn7 -- CellMonitoringUnit_3/LConn7
  CellMonitoringUnit_1/LConn15 -- Cell_Module_1/RConn15
  CellMonitoringUnit_1/LConn3 -- Cell_Module_1/RConn3
  Cell_Module_3/RConn12 -- CellMonitoringUnit_3/LConn12
  Cell_Module_2/RConn9 -- CellMonitoringUnit_2/LConn9
  CellMonitoringUnit_1/LConn11 -- Cell_Module_1/RConn11
  Cell_Module_3/RConn8 -- CellMonitoringUnit_3/LConn8
  Cell_Module_3/RConn2 -- CellMonitoringUnit_3/LConn2
  Cell_Module_3/RConn4 -- CellMonitoringUnit_3/LConn4
  Cell_Module_2/RConn2 -- CellMonitoringUnit_2/LConn2
  Cell_Module_2/RConn12 -- CellMonitoringUnit_2/LConn12
  Cell_Module_2/RConn16 -- CellMonitoringUnit_2/LConn16
  Cell_Module_2/RConn14 -- CellMonitoringUnit_2/LConn14
  Cell_Module_3/RConn3 -- CellMonitoringUnit_3/LConn3
  Cell_Module_2/RConn10 -- CellMonitoringUnit_2/LConn10
  CellMonitoringUnit_1/LConn7 -- Cell_Module_1/RConn7
  Cell+/RConn1 -- Cell_Module_1/RConn1 -- CellMonitoringUnit_2/LConn1 -- Cell_Module_2/RConn1 -- CellMonitoringUnit_3/LConn1 -- Cell_Module_3/RConn1 -- CellMonitoringUnit_1/LConn1
  Cell_Module_2/RConn8 -- CellMonitoringUnit_2/LConn8
  Cell_Module_2/RConn13 -- CellMonitoringUnit_2/LConn13
  CellMonitoringUnit_1/LConn8 -- Cell_Module_1/RConn8
  CellMonitoringUnit_1/LConn17 -- Cell_Module_2/RConn17 -- Cell_Module_3/RConn17 -- CellMonitoringUnit_3/LConn17 -- CellMonitoringUnit_2/LConn17 -- Cell-/RConn1 -- Cell_Module_1/RConn17
  Cell_Module_2/RConn6 -- CellMonitoringUnit_2/LConn6
  CellMonitoringUnit_1/LConn13 -- Cell_Module_1/RConn13
  Cell_Module_2/RConn5 -- CellMonitoringUnit_2/LConn5
  Cell_Module_3/RConn9 -- CellMonitoringUnit_3/LConn9
  Cell_Module_2/RConn11 -- CellMonitoringUnit_2/LConn11
  Cell_Module_3/RConn6 -- CellMonitoringUnit_3/LConn6
  CellMonitoringUnit_1/LConn9 -- Cell_Module_1/RConn9

== system Battery_Model/Battery_Pack/Battery_Pack_7Modules/Cell_3p06 ==
  BalCmd : Inport
  AmTmp : Inport  Port=2
  CellMonitoringUnit_1 : Subsystem
  CellMonitoringUnit_2 : Subsystem
  CellMonitoringUnit_3 : Subsystem
  Cell_Module_1 : Subsystem
  Cell_Module_2 : Subsystem
  Cell_Module_3 : Subsystem
  Data Type Conversion2 : DataTypeConversion  OutDataTypeStr=double
  Data Type Conversion3 : DataTypeConversion  OutDataTypeStr=single
  Data Type Conversion4 : DataTypeConversion  OutDataTypeStr=single
  Data Type Conversion5 : DataTypeConversion  OutDataTypeStr=single
  Vector Concatenate : Concatenate  NumInputs=3
  Vector Concatenate1 : Concatenate  NumInputs=3
  Cell+ : PMIOPort  Side=Right
  Cell- : PMIOPort  Port=2  Side=Right
  Cell_Voltages : Outport  VectorParamsAs1DForOutWhenUnconnected=off
  Cell_Temperatures : Outport  Port=2  VectorParamsAs1DForOutWhenUnconnected=off
  wires:
  Data Type Conversion4/1 -> [Module01_Volts]
  CellMonitoringUnit_1/1(CellVoltages) -> Data Type Conversion4/1
  Data Type Conversion2/1 -> CellMonitoringUnit_3/1(BalCmd), CellMonitoringUnit_2/1(BalCmd), CellMonitoringUnit_1/1(BalCmd)
  [Module01_Volts] -> Vector Concatenate/1  "Module01_Volts"
  Data Type Conversion5/1 -> [Module03_Volts]
  AmTmp/1 -> Cell_Module_3/1(AmbientTemp), Cell_Module_2/1(AmbientTemp), Cell_Module_1/1(AmbientTemp)
  CellMonitoringUnit_2/1(CellVoltages) -> Data Type Conversion3/1
  Data Type Conversion3/1 -> [Module02_Volts]
  Cell_Module_1/1(CellTemp) -> [Module01_Temps]
  Cell_Module_2/1(CellTemp) -> [Module02_Temps]
  BalCmd/1 -> Data Type Conversion2/1
  CellMonitoringUnit_3/1(CellVoltages) -> Data Type Conversion5/1
  [Module03_Volts] -> Vector Concatenate/3  "Module03_Volts"
  Vector Concatenate/1 -> Cell_Voltages/1
  [Module02_Volts] -> Vector Concatenate/2  "Module02_Volts"
  Cell_Module_3/1(CellTemp) -> [Module03_Temps]
  [Module03_Temps] -> Vector Concatenate1/3
  [Module01_Temps] -> Vector Concatenate1/1
  [Module02_Temps] -> Vector Concatenate1/2
  Vector Concatenate1/1 -> Cell_Temperatures/1
  connections:
  CellMonitoringUnit_1/LConn9 -- Cell_Module_1/RConn9
  Cell_Module_3/RConn6 -- CellMonitoringUnit_3/LConn6
  Cell_Module_2/RConn11 -- CellMonitoringUnit_2/LConn11
  Cell_Module_3/RConn9 -- CellMonitoringUnit_3/LConn9
  Cell_Module_2/RConn5 -- CellMonitoringUnit_2/LConn5
  CellMonitoringUnit_1/LConn13 -- Cell_Module_1/RConn13
  Cell_Module_2/RConn6 -- CellMonitoringUnit_2/LConn6
  Cell_Module_1/RConn17 -- Cell-/RConn1 -- CellMonitoringUnit_2/LConn17 -- CellMonitoringUnit_3/LConn17 -- Cell_Module_3/RConn17 -- Cell_Module_2/RConn17 -- CellMonitoringUnit_1/LConn17
  CellMonitoringUnit_1/LConn8 -- Cell_Module_1/RConn8
  Cell_Module_2/RConn13 -- CellMonitoringUnit_2/LConn13
  Cell_Module_2/RConn8 -- CellMonitoringUnit_2/LConn8
  CellMonitoringUnit_1/LConn1 -- Cell_Module_3/RConn1 -- CellMonitoringUnit_3/LConn1 -- Cell_Module_2/RConn1 -- CellMonitoringUnit_2/LConn1 -- Cell_Module_1/RConn1 -- Cell+/RConn1
  CellMonitoringUnit_1/LConn7 -- Cell_Module_1/RConn7
  Cell_Module_2/RConn10 -- CellMonitoringUnit_2/LConn10
  Cell_Module_3/RConn3 -- CellMonitoringUnit_3/LConn3
  Cell_Module_2/RConn14 -- CellMonitoringUnit_2/LConn14
  Cell_Module_2/RConn16 -- CellMonitoringUnit_2/LConn16
  Cell_Module_2/RConn12 -- CellMonitoringUnit_2/LConn12
  Cell_Module_2/RConn2 -- CellMonitoringUnit_2/LConn2
  Cell_Module_3/RConn4 -- CellMonitoringUnit_3/LConn4
  Cell_Module_3/RConn2 -- CellMonitoringUnit_3/LConn2
  Cell_Module_3/RConn8 -- CellMonitoringUnit_3/LConn8
  CellMonitoringUnit_1/LConn11 -- Cell_Module_1/RConn11
  Cell_Module_2/RConn9 -- CellMonitoringUnit_2/LConn9
  Cell_Module_3/RConn12 -- CellMonitoringUnit_3/LConn12
  CellMonitoringUnit_1/LConn3 -- Cell_Module_1/RConn3
  CellMonitoringUnit_1/LConn15 -- Cell_Module_1/RConn15
  Cell_Module_3/RConn7 -- CellMonitoringUnit_3/LConn7
  CellMonitoringUnit_1/LConn5 -- Cell_Module_1/RConn5
  Cell_Module_3/RConn15 -- CellMonitoringUnit_3/LConn15
  CellMonitoringUnit_1/LConn12 -- Cell_Module_1/RConn12
  CellMonitoringUnit_1/LConn10 -- Cell_Module_1/RConn10
  Cell_Module_2/RConn3 -- CellMonitoringUnit_2/LConn3
  CellMonitoringUnit_1/LConn6 -- Cell_Module_1/RConn6
  Cell_Module_2/RConn4 -- CellMonitoringUnit_2/LConn4
  Cell_Module_3/RConn10 -- CellMonitoringUnit_3/LConn10
  CellMonitoringUnit_1/LConn14 -- Cell_Module_1/RConn14
  CellMonitoringUnit_1/LConn4 -- Cell_Module_1/RConn4
  Cell_Module_3/RConn16 -- CellMonitoringUnit_3/LConn16
  Cell_Module_3/RConn11 -- CellMonitoringUnit_3/LConn11
  Cell_Module_3/RConn13 -- CellMonitoringUnit_3/LConn13
  Cell_Module_3/RConn14 -- CellMonitoringUnit_3/LConn14
  Cell_Module_3/RConn5 -- CellMonitoringUnit_3/LConn5
  Cell_Module_2/RConn15 -- CellMonitoringUnit_2/LConn15
  Cell_Module_2/RConn7 -- CellMonitoringUnit_2/LConn7
  CellMonitoringUnit_1/LConn2 -- Cell_Module_1/RConn2
  CellMonitoringUnit_1/LConn16 -- Cell_Module_1/RConn16
